simulink model "lotka_volterra"  (R2023a)
settings: Solver=VariableStepAuto  StartTime=0.0  StopTime=100  RelTol=1e-3
settings Model: Creator=ramir  LastModifiedBy=ramir
settings DataIOCC: ReturnWorkspaceOutputs=off  TimeSaveName=t

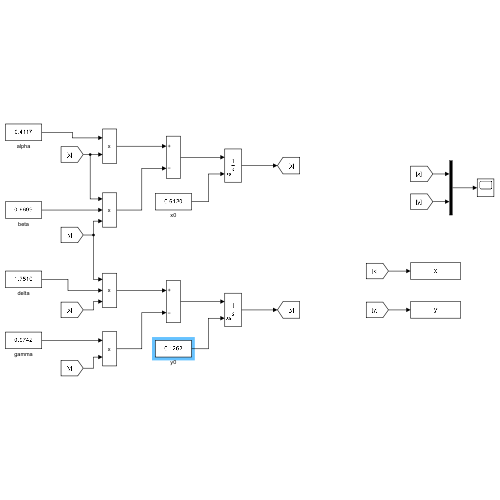
[thumbnail: Simulink's stored preview of the top-level diagram]
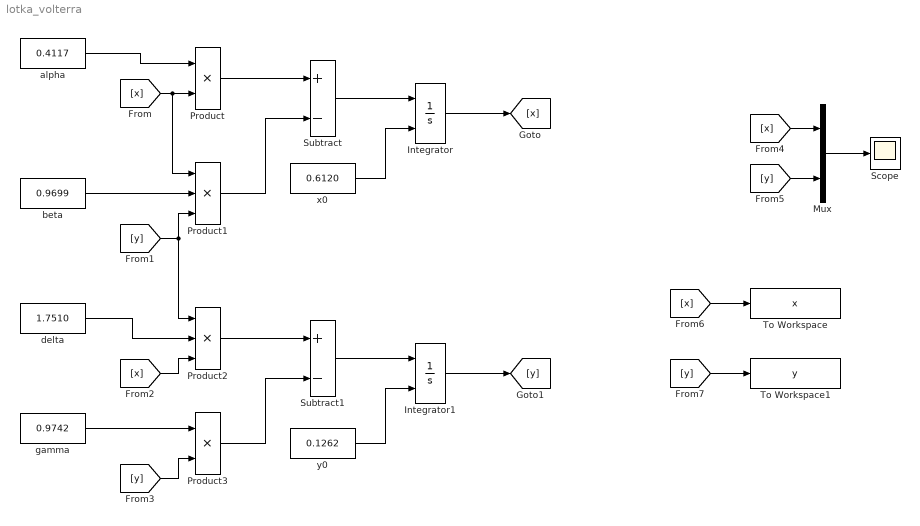
== system lotka_volterra ==
  Integrator : Integrator  InitialConditionSource=external
  Integrator1 : Integrator  InitialConditionSource=external
  Mux : Mux  Inputs=2
  Product : Product
  Product1 : Product  Inputs=3
  Product2 : Product  Inputs=3
  Product3 : Product
  Scope : Scope
  Subtract : Sum  Inputs=+-
  Subtract1 : Sum  Inputs=+-
  To Workspace : ToWorkspace  VariableName=x  SampleTime=-1
  To Workspace1 : ToWorkspace  VariableName=y  SampleTime=-1
  alpha : Constant  Value=0.4117
  beta : Constant  Value=0.9699
  delta : Constant  Value=1.7510
  gamma : Constant  Value=0.9742
  x0 : Constant  Value=0.6120
  y0 : Constant  Value=0.1262
  wires:
  alpha/1 -> Product/1
  [x] -> Product1/1, Product/2
  beta/1 -> Product1/2
  [y] -> Product2/1, Product1/3
  delta/1 -> Product2/2
  gamma/1 -> Product3/1
  [x] -> Product2/3
  [y] -> Product3/2
  Subtract1/1 -> Integrator1/1
  Product/1 -> Subtract/1
  Product1/1 -> Subtract/2
  Subtract/1 -> Integrator/1
  x0/1 -> Integrator/2
  Product2/1 -> Subtract1/1
  Product3/1 -> Subtract1/2
  y0/1 -> Integrator1/2
  Integrator/1 -> [x]
  Integrator1/1 -> [y]
  [x] -> Mux/1
  [y] -> Mux/2
  Mux/1 -> Scope/1
  [x] -> To Workspace/1
  [y] -> To Workspace1/1
